simulink model "mdaqdemo_usend"  (R2014b)
settings: Solver=FixedStepDiscrete  SolverMode=SingleTasking  StartTime=0.0  StopTime=10.0  FixedStep=0.1  RelTol=1e-3
libraries: etargetslib x1
settings Model: Creator=peselnikmg  LastModifiedBy=peselnikmg
settings OptimizationCC: OptimizeModelRefInitCode=on  LifeSpan=1
settings DebuggingCC: UnderspecifiedInitializationDetection=Classic  MergeDetectMultiDrivingBlocksExec=none
settings HardwareCC: ProdBitPerLong=40  ProdLargestAtomicInteger=Integer  ProdIntDivRoundTo=Zero  ProdEndianess=LittleEndian  ProdHWDeviceType=Texas Instruments->C6000
settings RTWCC: SystemTargetFile=microdaq.tlc  TemplateMakefile=microdaq.tmf  PostCodeGenCommand=microdaq_postcodegen(buildInfo)  Description=MicroDAQ Real-Time Measurement System  GenerateReport=on  ProcessScript=microdaq_make_rtw_hook  IncludeHyperlinkInReport=on  LaunchReport=on  GenerateTraceInfo=on  GenerateTraceReport=on  GenerateTraceReportSl=on  GenerateTraceReportSf=on  GenerateTraceReportEml=on
settings CodeAppCC: IgnoreCustomStorageClasses=off
settings STFCustomTargetCC: CodeReplacementLibrary=TI C674x  CombineOutputUpdateFcns=on  ERTCustomFileBanners=on  SupportContinuousTime=off  SupportNonInlinedSFcns=off  MATLABClassNameForMDSCustomization=Simulink.SoftwareTarget.ERTCustomization  GRTInterface=off  SystemTargetFile=microdaq.tlc
settings ERTTargetCC: CodeReplacementLibrary=TI C674x  ParMdlRefBuildCompliant=off  CompOptLevelCompliant=off  ConcurrentExecutionCompliant=off  ERTFirstTimeCompliant=off  ModelStepFunctionPrototypeControlCompliant=off  CPPClassGenCompliant=off  ExtModeStaticAlloc=on  ExtModeStaticAllocSize=10485760  ExtModeMexArgs=getpref('microdaq','TargetIP') 1 4344  InlinedParameterPlacement=NonHierarchical  ERTCustomFileTemplate=microdaq_main.tlc

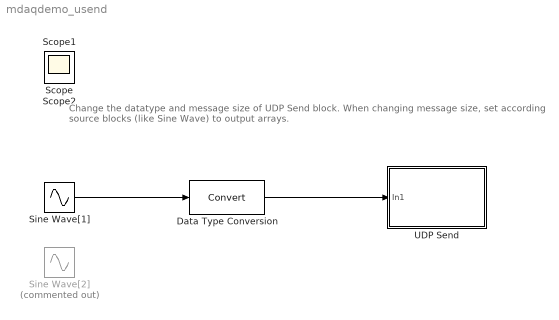
== system mdaqdemo_usend ==
  note: Change the datatype and message size of UDP Send block.
      | When changing message size, set according source blocks (like Sine Wave) to output arrays.
  Data Type Conversion : DataTypeConversion
  Sine Wave[1] : Sin
  Sine Wave[2] : Sin  Commented=on  Amplitude=[1 2]
  UDP Send : Subsystem  mask(UDP Send){IPAddrStr='10.10.1.10', Port=5000, Blocking=off, Timeout=250, Datatype=double, SizePack=1, SampleTime=-1}
      mask prompts: IPAddrStr "Remote IP address:"; Port "Remote port:"; Timeout "Timeout (ms):"; Datatype "Data type:"; SizePack "Message size (in data type units):"; SampleTime "Sample time:"
      mask help: Send UDP packets to given IP port and address.
      mask init:
      | % Convert string IP Address to bytes
      | % for use in S-function
      | IPAddr = double(IPAddrStr);
      | % UDP Protocol
      | Protocol = 1;
      | % Construct data type expression for Pack block
      | %packdt = repmat({Datatype},SizePack,1);
      | packdt = {Datatype};
      | % Any better way to find data type size?
      | eval(['dummy = ',Datatype,'(0);']);
      | dummy = whos('dummy');
      | Size = SizePack*dummy.bytes;
      mask TypeOptions Datatype: double | single | uint8 | uint16 | uint32 | int8 | int16 | int32 | boolean
      mask Display:
      | color('blue');
      | text(0.98, 0.13, 'MicroDAQ', 'horizontalalignment', 'right');
      | color('black');
      | fprintf('UDP Send\n\n\n');
      | color('gray');
  Scope : Scope
  Scope1 : Scope
  Scope2 : Scope
      settings: SaveName=ScopeData2
  wires:
  Data Type Conversion/1 -> UDP Send/1(In1)
  Sine Wave[1]/1 -> Data Type Conversion/1

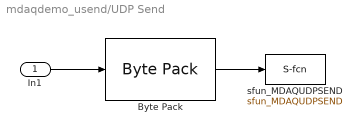
== system mdaqdemo_usend/UDP Send ==
  In1 : Inport  PortDimensions=SizePack
  Byte Pack : etargetslib/Byte Pack  datatypes=packdt  byteAlign=1
  sfun_MDAQUDPSEND : S-Function  FunctionName=sfun_MDAQUDPSEND  Parameters=IPAddr, Port, Blocking, Timeout, Protocol, Size, SampleTime  EnableBusSupport=off
  wires:
  Byte Pack/1 -> sfun_MDAQUDPSEND/1
  In1/1 -> Byte Pack/1
